simulink model "Impedance_based_model"  (R2016b)
settings: Solver=VariableStepAuto  StartTime=0.0  StopTime=1  RelTol=1e-3
libraries: powerlib x12, aerolibconvert2 x5, powerlib_meascontrol x4
settings Model: Creator=Neel  LastModifiedBy=Neel

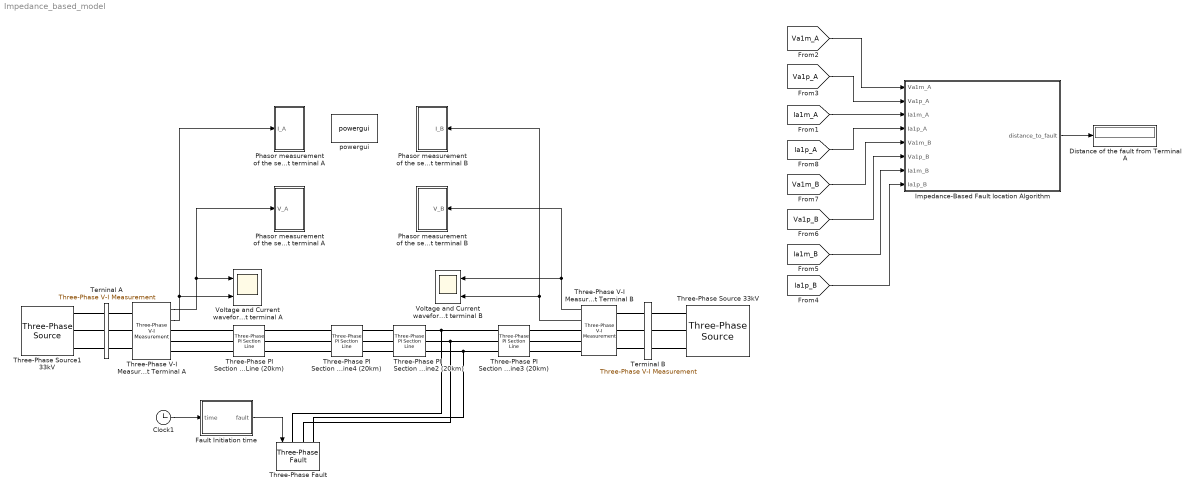
== system Impedance_based_model ==
  Clock1 : Clock
  Distance of the fault from Terminal A : Display
  Fault Initiation time : MATLAB Function  TreatAsAtomicUnit=on
  Impedance-Based Fault location Algorithm : MATLAB Function  TreatAsAtomicUnit=on
  Phasor measurement of the sequence currents at terminal A : Subsystem
  Phasor measurement of the sequence currents at terminal B : Subsystem
  Phasor measurement of the sequence voltages at terminal A : Subsystem
  Phasor measurement of the sequence voltages at terminal B : Subsystem
  Terminal B : powerlib/Measurements/Three-Phase V-I Measurement  VoltageMeasurement=no  SetLabelV=off  LabelV=Vabc  Vpu=off  VpuLL=off  CurrentMeasurement=no  SetLabelI=off  LabelI=Iabc  Ipu=off  Pbase=100e6  Vbase=500e3  OutputType=Complex  PhasorSimulation=off  PSBequivalent=0
  Terninal A : powerlib/Measurements/Three-Phase V-I Measurement  VoltageMeasurement=no  SetLabelV=off  LabelV=Vabc  Vpu=off  VpuLL=off  CurrentMeasurement=no  SetLabelI=off  LabelI=Iabc  Ipu=off  Pbase=100e6  Vbase=500e3  OutputType=Complex  PhasorSimulation=off  PSBequivalent=0
  Three-Phase PI Section Line (20km) : powerlib/Elements/Three-Phase PI Section Line  LConnTagsString=a|b|c  RConnTagsString=A|B|C  Frequency=50  Resistances=[ 0.01273 0.3864]  Inductances="[ 0.9337e-3  4.1264e-3]"  Capacitances=[12.74e-9 7.751e-9]  Length=20
  Three-Phase PI Section Line2 (20km) : powerlib/Elements/Three-Phase PI Section Line  LConnTagsString=a|b|c  RConnTagsString=A|B|C  Frequency=50  Resistances=[ 0.01273 0.3864]  Inductances="[ 0.9337e-3  4.1264e-3]"  Capacitances=[12.74e-9 7.751e-9]  Length=20
  Three-Phase PI Section Line3 (20km) : powerlib/Elements/Three-Phase PI Section Line  LConnTagsString=a|b|c  RConnTagsString=A|B|C  Frequency=50  Resistances=[ 0.01273 0.3864]  Inductances="[ 0.9337e-3  4.1264e-3]"  Capacitances=[12.74e-9 7.751e-9]  Length=20
  Three-Phase PI Section Line4 (20km) : powerlib/Elements/Three-Phase PI Section Line  LConnTagsString=a|b|c  RConnTagsString=A|B|C  Frequency=50  Resistances=[ 0.01273 0.3864]  Inductances="[ 0.9337e-3  4.1264e-3]"  Capacitances=[12.74e-9 7.751e-9]  Length=20
  Three-Phase V-I Measurement at Terminal A : powerlib/Measurements/Three-Phase V-I Measurement  VoltageMeasurement=phase-to-ground  SetLabelV=off  LabelV=Vabc  Vpu=on  VpuLL=off  CurrentMeasurement=yes  SetLabelI=off  LabelI=Iabc  Ipu=off  Pbase=1e6  Vbase=11e3  OutputType=Magnitude  PhasorSimulation=off  PSBequivalent=0
  Three-Phase V-I Measurement at Terminal B : powerlib/Measurements/Three-Phase V-I Measurement  VoltageMeasurement=phase-to-ground  SetLabelV=off  LabelV=Vabc  Vpu=on  VpuLL=off  CurrentMeasurement=yes  SetLabelI=off  LabelI=Iabc  Ipu=off  Pbase=1e6  Vbase=11e3  OutputType=Magnitude  PhasorSimulation=off  PSBequivalent=0
  Three-Phase Fault : powerlib/Elements/Three-Phase Fault  InitialStates=0  FaultA=on  FaultB=off  FaultC=off  GroundFault=on  SwitchTimes="[1/60  5/60]"  External=on  SwitchStatus=NaN  FaultResistance=0.001  GroundResistance=0.01  SnubberResistance=1e6  SnubberCapacitance=inf  Measurements=None
  Three-Phase Source 33kV : powerlib/Electrical Sources/Three-Phase Source  InternalConnection=Yg  VoltagePhases=off  Voltage=33e3  PhaseAngle=-20  Voltage_phases=[25e3 25e3 25e3]/sqrt(3)  PhaseAngles_phases=[0 -120 +120]  Frequency=50  NonIdealSource=on  SpecifyImpedance=off  Resistance=0.8929  Inductance=16.58e-3  ShortCircuitLevel=100e6  BaseVoltage=33e3  XRratio=7  BusType=swing  Pref=10e3  Qref=0  Prefabc=[10e3, 10e3, 10e3]  Qrefabc=[0, 0, 0]  Qmin=-inf  Qmax=inf
  Three-Phase Source1 33kV : powerlib/Electrical Sources/Three-Phase Source  InternalConnection=Yg  VoltagePhases=off  Voltage=33e3  PhaseAngle=0  Voltage_phases=[25e3 25e3 25e3]/sqrt(3)  PhaseAngles_phases=[0 -120 +120]  Frequency=50  NonIdealSource=on  SpecifyImpedance=off  Resistance=0.8929  Inductance=16.58e-3  ShortCircuitLevel=100e6  BaseVoltage=33e3  XRratio=7  BusType=swing  Pref=10e3  Qref=0  Prefabc=[10e3, 10e3, 10e3]  Qrefabc=[0, 0, 0]  Qmin=-inf  Qmax=inf
  Voltage and Current waveform at terminal A : Scope  NumInputPorts=2
  Voltage and Current waveform at terminal B : Scope  NumInputPorts=2
  powergui : powerlib/powergui  Priority=1  SimulationMode=Discrete  SolverType=Tustin/Backward Euler (TBE)  SampleTime=8e-5  frequency=50  SPID=off  DisableSnubberDevices=off  DisableRonSwitches=off  DisableVfSwitches=off  SwTol=0  DisplayEquations=off  Interpol=off  ExternalGateDelay=off  methode=off  Ts=10  FunctionMessages=off  echomessages=off  HookPort=off  EnableUseOfTLC=off  x0status=blocks  frequencyindice=50  Pbase=100e6  ErrMax=1e-4  Iterations=50  UnitsV=kV  UnitsW=MW  buscounter=0  RestoreLinks=warning  ResistiveCurrentMeasurement=off  Frange=[0:2:500]  Ylog=off  Xlog=on  ShowGrid=off  save=off  variable=ZData  structure=0  ZoomFFT=off  StartTime=0.0  cycles=1  DisplayStyle=1  fundamental=60  FreqAxis=off  MaxFrequency=1000  frequencyindicesteady=1  RmsSteady=1  display=off
  wires:
  Three-Phase V-I Measurement at Terminal A/2 -> Phasor measurement of the sequence currents at terminal A/1(I_A), Voltage and Current waveform at terminal A/2
  Three-Phase V-I Measurement at Terminal B/2 -> Phasor measurement of the sequence currents at terminal B/1(I_B), Voltage and Current waveform at terminal B/2
  Clock1/1 -> Fault Initiation time/1(time)
  Fault Initiation time/1(fault) -> Three-Phase Fault/1
  Three-Phase V-I Measurement at Terminal B/1 -> Voltage and Current waveform at terminal B/1, Phasor measurement of the sequence voltages at terminal B/1(V_B)
  Three-Phase V-I Measurement at Terminal A/1 -> Phasor measurement of the sequence voltages at terminal A/1(V_A), Voltage and Current waveform at terminal A/1
  [Va1m_A] -> Impedance-Based Fault location Algorithm/1(Va1m_A)
  [Va1p_A] -> Impedance-Based Fault location Algorithm/2(Va1p_A)
  [Ia1m_A] -> Impedance-Based Fault location Algorithm/3(Ia1m_A)
  [Ia1p_A] -> Impedance-Based Fault location Algorithm/4(Ia1p_A)
  [Va1m_B] -> Impedance-Based Fault location Algorithm/5(Va1m_B)
  [Va1p_B] -> Impedance-Based Fault location Algorithm/6(Va1p_B)
  [Ia1m_B] -> Impedance-Based Fault location Algorithm/7(Ia1m_B)
  [Ia1p_B] -> Impedance-Based Fault location Algorithm/8(Ia1p_B)
  Impedance-Based Fault location Algorithm/1(distance_to_fault) -> Distance of the fault from Terminal A/1
  connections:
  Terminal B/LConn3 -- Three-Phase V-I Measurement at Terminal B/LConn3
  Terminal B/LConn2 -- Three-Phase V-I Measurement at Terminal B/LConn2
  Three-Phase Source 33kV/RConn2 -- Terminal B/RConn2
  Three-Phase PI Section Line3 (20km)/RConn1 -- Three-Phase V-I Measurement at Terminal B/RConn1
  Terninal A/RConn3 -- Three-Phase V-I Measurement at Terminal A/LConn3
  Three-Phase Source1 33kV/RConn1 -- Terninal A/LConn1
  Three-Phase PI Section Line3 (20km)/LConn2 -- Three-Phase Fault/LConn2 -- Three-Phase PI Section Line2 (20km)/RConn2
  Three-Phase PI Section Line4 (20km)/RConn2 -- Three-Phase PI Section Line2 (20km)/LConn2
  Three-Phase PI Section Line3 (20km)/LConn3 -- Three-Phase Fault/LConn3 -- Three-Phase PI Section Line2 (20km)/RConn3
  Three-Phase Source 33kV/RConn3 -- Terminal B/RConn3
  Three-Phase PI Section Line3 (20km)/LConn1 -- Three-Phase Fault/LConn1 -- Three-Phase PI Section Line2 (20km)/RConn1
  Three-Phase Source 33kV/RConn1 -- Terminal B/RConn1
  Three-Phase PI Section Line4 (20km)/RConn3 -- Three-Phase PI Section Line2 (20km)/LConn3
  Three-Phase PI Section Line4 (20km)/RConn1 -- Three-Phase PI Section Line2 (20km)/LConn1
  Three-Phase PI Section Line3 (20km)/RConn2 -- Three-Phase V-I Measurement at Terminal B/RConn2
  Three-Phase PI Section Line (20km)/LConn1 -- Three-Phase V-I Measurement at Terminal A/RConn1
  Terminal B/LConn1 -- Three-Phase V-I Measurement at Terminal B/LConn1
  Three-Phase Source1 33kV/RConn3 -- Terninal A/LConn3
  Terninal A/RConn1 -- Three-Phase V-I Measurement at Terminal A/LConn1
  Terninal A/RConn2 -- Three-Phase V-I Measurement at Terminal A/LConn2
  Three-Phase Source1 33kV/RConn2 -- Terninal A/LConn2
  Three-Phase PI Section Line3 (20km)/RConn3 -- Three-Phase V-I Measurement at Terminal B/RConn3
  Three-Phase PI Section Line (20km)/LConn3 -- Three-Phase V-I Measurement at Terminal A/RConn3
  Three-Phase PI Section Line (20km)/LConn2 -- Three-Phase V-I Measurement at Terminal A/RConn2
  Three-Phase PI Section Line4 (20km)/LConn1 -- Three-Phase PI Section Line (20km)/RConn1
  Three-Phase PI Section Line4 (20km)/LConn2 -- Three-Phase PI Section Line (20km)/RConn2
  Three-Phase PI Section Line4 (20km)/LConn3 -- Three-Phase PI Section Line (20km)/RConn3

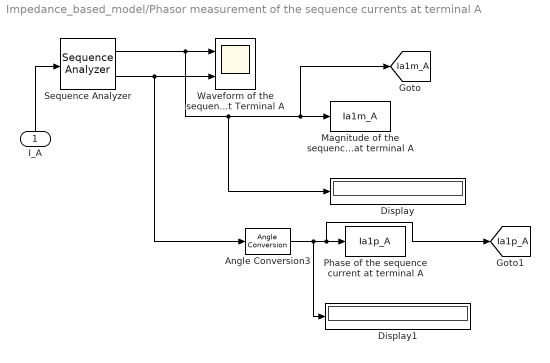
== system Impedance_based_model/Phasor measurement of the sequence currents at terminal A ==
  I_A : Inport
  Angle Conversion3 : aerolibconvert2/Angle Conversion  IU=deg  OU=rad
  Display : Display
  Display1 : Display
  Magnitude of the sequence current at terminal A : ToWorkspace  VariableName=Ia1m_A  SampleTime=-1
  Phase of the sequence current at terminal A : ToWorkspace  VariableName=Ia1p_A  SampleTime=-1
  Sequence Analyzer : powerlib_meascontrol/Measurements/Sequence Analyzer  Freq=50  n=1  seq=Negative  InInit=[1, 0]  Ts=0
  Waveform of the sequence current at Terminal A : Scope  NumInputPorts=2
  tag scope: Ia1m_A=global, Ia1p_A=global
  wires:
  I_A/1 -> Sequence Analyzer/1
  Angle Conversion3/1 -> Display1/1, [Ia1p_A], Phase of the sequence current at terminal A/1
  Sequence Analyzer/1 -> Display/1, [Ia1m_A], Magnitude of the sequence current at terminal A/1, Waveform of the sequence current at Terminal A/1
  Sequence Analyzer/2 -> Angle Conversion3/1, Waveform of the sequence current at Terminal A/2

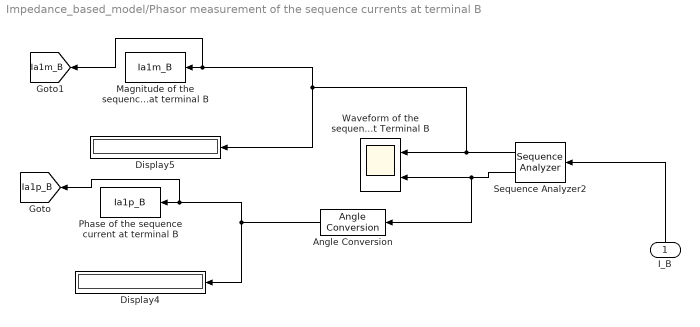
== system Impedance_based_model/Phasor measurement of the sequence currents at terminal B ==
  I_B : Inport
  Angle Conversion : aerolibconvert2/Angle Conversion  IU=deg  OU=rad
  Display4 : Display
  Display5 : Display
  Magnitude of the sequence current at terminal B : ToWorkspace  VariableName=Ia1m_B  SampleTime=-1
  Phase of the sequence current at terminal B : ToWorkspace  VariableName=Ia1p_B  SampleTime=-1
  Sequence Analyzer2 : powerlib_meascontrol/Measurements/Sequence Analyzer  Freq=50  n=1  seq=Negative  InInit=[1, 0]  Ts=0
  Waveform of the sequence current at Terminal B : Scope  NumInputPorts=2
  tag scope: Ia1m_B=global, Ia1p_B=global
  wires:
  I_B/1 -> Sequence Analyzer2/1
  Sequence Analyzer2/2 -> Angle Conversion/1, Waveform of the sequence current at Terminal B/2
  Angle Conversion/1 -> Display4/1, [Ia1p_B], Phase of the sequence current at terminal B/1
  Sequence Analyzer2/1 -> Display5/1, [Ia1m_B], Magnitude of the sequence current at terminal B/1, Waveform of the sequence current at Terminal B/1

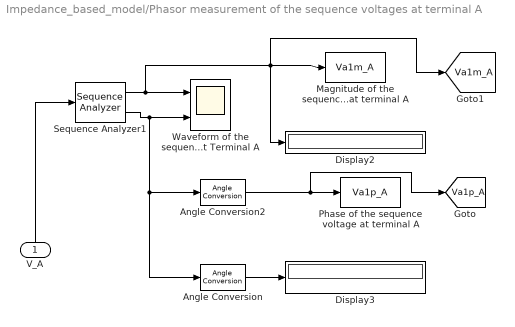
== system Impedance_based_model/Phasor measurement of the sequence voltages at terminal A ==
  V_A : Inport
  Angle Conversion : aerolibconvert2/Angle Conversion  IU=deg  OU=rad
  Angle Conversion2 : aerolibconvert2/Angle Conversion  IU=deg  OU=rad
  Display2 : Display
  Display3 : Display
  Magnitude of the sequence voltage at terminal A : ToWorkspace  VariableName=Va1m_A  SampleTime=-1
  Phase of the sequence voltage at terminal A : ToWorkspace  VariableName=Va1p_A  SampleTime=-1
  Sequence Analyzer1 : powerlib_meascontrol/Measurements/Sequence Analyzer  Freq=50  n=1  seq=Negative  InInit=[1, 0]  Ts=0
  Waveform of the sequence voltage at Terminal A : Scope  NumInputPorts=2
  tag scope: Va1m_A=global, Va1p_A=global
  wires:
  V_A/1 -> Sequence Analyzer1/1
  Angle Conversion/1 -> Display3/1
  Angle Conversion2/1 -> [Va1p_A], Phase of the sequence voltage at terminal A/1
  Sequence Analyzer1/1 -> Display2/1, Magnitude of the sequence voltage at terminal A/1, [Va1m_A], Waveform of the sequence voltage at Terminal A/1
  Sequence Analyzer1/2 -> Angle Conversion/1, Angle Conversion2/1, Waveform of the sequence voltage at Terminal A/2

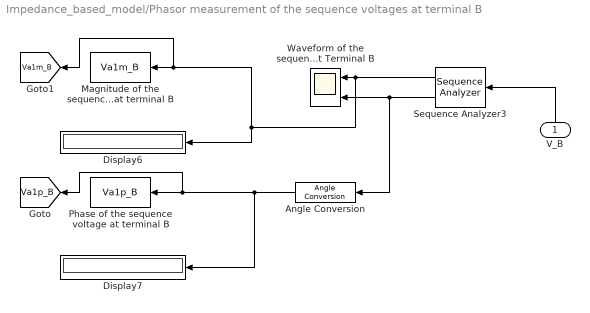
== system Impedance_based_model/Phasor measurement of the sequence voltages at terminal B ==
  V_B : Inport
  Angle Conversion : aerolibconvert2/Angle Conversion  IU=deg  OU=rad
  Display6 : Display
  Display7 : Display
  Magnitude of the sequence voltage at terminal B : ToWorkspace  VariableName=Va1m_B  SampleTime=-1
  Phase of the sequence voltage at terminal B : ToWorkspace  VariableName=Va1p_B  SampleTime=-1
  Sequence Analyzer3 : powerlib_meascontrol/Measurements/Sequence Analyzer  Freq=50  n=1  seq=Negative  InInit=[1, 0]  Ts=0
  Waveform of the sequence voltage at Terminal B : Scope  NumInputPorts=2
  tag scope: Va1m_B=global, Va1p_B=global
  wires:
  V_B/1 -> Sequence Analyzer3/1
  Sequence Analyzer3/1 -> [Va1m_B], Magnitude of the sequence voltage at terminal B/1, Display6/1, Waveform of the sequence voltage at Terminal B/1
  Sequence Analyzer3/2 -> Angle Conversion/1, Waveform of the sequence voltage at Terminal B/2
  Angle Conversion/1 -> [Va1p_B], Phase of the sequence voltage at terminal B/1, Display7/1

== matlab function Impedance_based_model/Impedance-Based Fault location Algorithm ==
  data: Va1m_A input; distance_to_fault output; Va1p_A input; Ia1m_A input; Ia1p_A input; Va1m_B input; Va1p_B input; Ia1m_B input; Ia1p_B input
% DESIGN AND TESTING OF SMART FAULT LOCATION ALGORITHMS FOR SMART
%                   TRANSMISSION AND DISTRIBUTION GRIDS

% ************************ BSc Electrical Engineering *******************

% ************************* Ramseebaluck Neelesh ************************
% *************************       RMSNEE002      ************************
% ************************* University of Cape Town *********************

function distance_to_fault = fcn(Va1m_A, Va1p_A, Ia1m_A, Ia1p_A, Va1m_B, Va1p_B, Ia1m_B, Ia1p_B)

line_length = 80;
R= 0.01273;         %pu resistance of transmission line
X= 0.0009337;       %pu inductance of transmission line

%...Acquiring the sequence voltage and current values at both
%terminals...%
% For terminal A
a1= Va1m_A;          %magnitude of voltage at Bus A
b1= Va1p_A;          %voltage phase at Bus A
a2= Ia1m_A;          %current magnitude at Bus A
b2= Ia1p_A;          %current phase at Bus A
% For terminal B
a3= Va1m_B;          %magnitude of voltage at Bus B
b3= Va1p_B;          %voltage phase at Bus B
a4= Ia1m_B;          %current magnitude at Bus B
b4= Ia1p_B;          %current phase at Bus B

% Calculation of the coefficients 
coeff1= R*a2 - X*b2;                  %coefficient1
coeff2= R*b2 + X*a2;                 %coefficient2
coeff3= R*a4 - X*b4;                 %coefficient3
coeff4= R*b4 + X*a4;                 %coefficient4

% Solving(A1)sin(delta) + (A2)cos(delta)+ A3 = 0

A1 = (-coeff3*a1)-(coeff4*b1)-(coeff1*a3)-(coeff2*b3)+(coeff1*coeff3)+(coeff2*coeff4);
A2 = (coeff4*a1)-(coeff3*b1)-(coeff2*a3)+(coeff1*b3)+(coeff2*coeff3)-(coeff1*coeff4);
A3 = (coeff2*a1)-(coeff1*b1)-(coeff4*a3)+(coeff3*b3);

%Applying the Newton- Raphson's Method

delta = zeros(30,1);                  % Synchronization angle at k iteration
New_delta = zeros (31, 1);            % Synchronization angle at k+1 iteration

New_delta (1) = 0;                    % Initial guess for the synchronization angle

for k= 1:30
delta(k)= New_delta(k);
% Solving the iterative equations...equation(5.21)
f1 = A2*cos(delta(k)) +A1*sin(delta(k)) + A3;
f2 = A1*cos(delta(k))-A2*sin(delta(k));

New_delta (k+1) = delta(k)-(f1/f2);
%difference= abs(New_delta(k+1)-delta(k));
%Calculating the per unit distance m using equation(5.24)
distance_m =(a1*sin(New_delta(k+1))+b1*cos(New_delta(k+1))-b3+coeff4)/(coeff1*sin(New_delta(k+1))+coeff2*cos(New_delta(k+1))+coeff4);

%fault distance from terminal A.
distance_to_fault = distance_m * line_length;

end

== matlab function Impedance_based_model/Fault Initiation time ==
  data: time input; fault output
function fault = fcn(time)
%#codegen
fault=0;
if (time>=0.2)
    fault=1;
end
